simulink model "torque_to_theta"  (R2018b)
settings: Solver=FixedStepAuto  StartTime=0.0  StopTime=inf  RelTol=1e-3
values from neighbouring files (symbols this model uses):
  p = pi    (= 3.14159265359)    [nominal_model.m]
libraries: arduinolib x15, simulink x3
settings Model: ExtModeTrigDuration=2  Creator=paniz  LastModifiedBy=paniz
settings DataIOCC: ReturnWorkspaceOutputs=on
settings OptimizationCC: EnhancedBackFolding=on  PassReuseOutputArgsAs=Individual arguments  ZeroExternalMemoryAtStartup=off  ZeroInternalMemoryAtStartup=off  MaxStackSize=64  OptimizeBlockOrder=speed  DifferentSizesBufferReuse=on  OptimizationCustomize=off
settings DebuggingCC: ParameterTunabilityLossMsg=error  UnconnectedInputMsg=none  UnconnectedOutputMsg=none  UnconnectedLineMsg=none  SFMachineParentedDataDiag=error
settings HardwareCC: ProdBitPerInt=16  ProdBitPerPointer=16  ProdBitPerSizeT=16  ProdBitPerPtrDiffT=16  ProdLargestAtomicFloat=None  ProdWordSize=8  ProdHWDeviceType=Atmel->AVR
settings SFSimCC: MATLABDynamicMemAlloc=off
settings RTWCC: SystemTargetFile=ert.tlc  HardwareBoard=Arduino Mega 2560  TemplateMakefile=ert_default_tmf  Toolchain=Arduino AVR
settings CodeAppCC: ForceParamTrailComments=on  IgnoreCustomStorageClasses=off  OperatorAnnotations=on  SimulinkDataObjDesc=on  SFDataObjDesc=on  InsertBlockDesc=on
settings ERTTargetCC: SupportContinuousTime=on  SupportVariableSizeSignals=on  ExtMode=on  ExtModeTransport=3  ExtModeStaticAlloc=on  ExtModeStaticAllocSize=2048  ExtModeMexFile=ext_xcp  ExtModeMexArgs=0 5 921600 'C:\Users\paniz\myCodes\Using Arduino and Matlab\Codes\Simulink\3 Muscle with pressure regulator\untitled.elf' 3 1000  ExtModeIntrfLevel=Level2 - Open

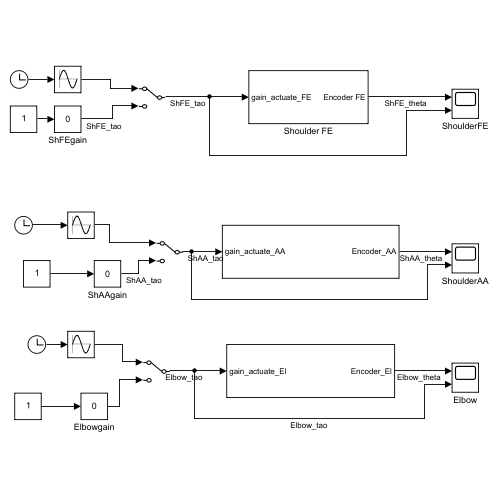
[thumbnail: Simulink's stored preview of the top-level diagram]
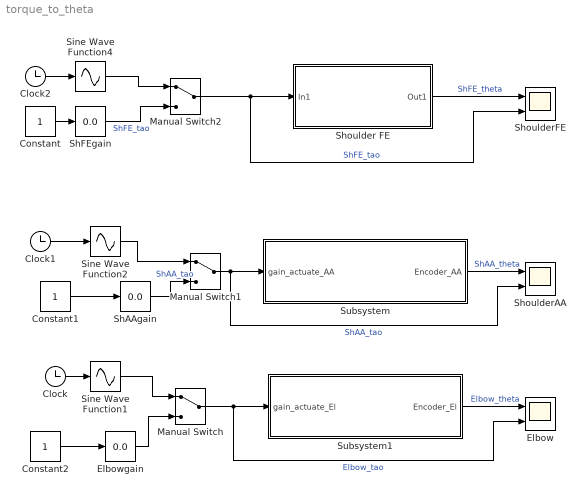
== system torque_to_theta ==
  Clock : Clock
  Clock1 : Clock
  Clock2 : Clock
  Constant : Constant
  Constant1 : Constant
  Constant2 : Constant
  Elbow : Scope  NumInputPorts=2
  Elbowgain : simulink/Math Operations/Slider Gain  gain=0.0  low=0  high=6
  Manual Switch : ManualSwitch
  Manual Switch1 : ManualSwitch
  Manual Switch2 : ManualSwitch
  ShAAgain : simulink/Math Operations/Slider Gain  gain=0.0  low=0  high=6
  ShFEgain : simulink/Math Operations/Slider Gain  gain=0.0  low=0  high=6
  Shoulder FE : Subsystem
  ShoulderAA : Scope  NumInputPorts=2
  ShoulderFE : Scope  NumInputPorts=2
  Sine Wave Function1 : Sin  TimeSource=Use external signal  Amplitude=2.3  Bias=2.30  Frequency=1/50  SampleTime=0
  Sine Wave Function2 : Sin  TimeSource=Use external signal  Amplitude=3  Bias=3  Frequency=1/50  Phase=-pi/3  SampleTime=0
  Sine Wave Function4 : Sin  TimeSource=Use external signal  Amplitude=3  Bias=3  Frequency=1/50  Phase=pi/6  SampleTime=0
  Subsystem : Subsystem
  Subsystem1 : Subsystem
  wires:
  Constant/1 -> ShFEgain/1
  ShFEgain/1 -> Manual Switch2/2  "ShFE_tao"
  Shoulder FE/1(Out1) -> ShoulderFE/1  "ShFE_theta"
  Manual Switch/1 -> Elbow/2, Subsystem1/1(gain_actuate_El)  "Elbow_tao"
  Subsystem1/1(Encoder_El) -> Elbow/1  "Elbow_theta"
  Subsystem/1(Encoder_AA) -> ShoulderAA/1  "ShAA_theta"
  Constant1/1 -> ShAAgain/1
  Constant2/1 -> Elbowgain/1
  Elbowgain/1 -> Manual Switch/2
  Sine Wave Function1/1 -> Manual Switch/1
  Clock/1 -> Sine Wave Function1/1
  Clock1/1 -> Sine Wave Function2/1
  Sine Wave Function2/1 -> Manual Switch1/1
  Manual Switch1/1 -> ShoulderAA/2, Subsystem/1(gain_actuate_AA)  "ShAA_tao"
  ShAAgain/1 -> Manual Switch1/2  "ShAA_tao"
  Clock2/1 -> Sine Wave Function4/1
  Sine Wave Function4/1 -> Manual Switch2/1
  Manual Switch2/1 -> ShoulderFE/2, Shoulder FE/1(In1)  "ShFE_tao"

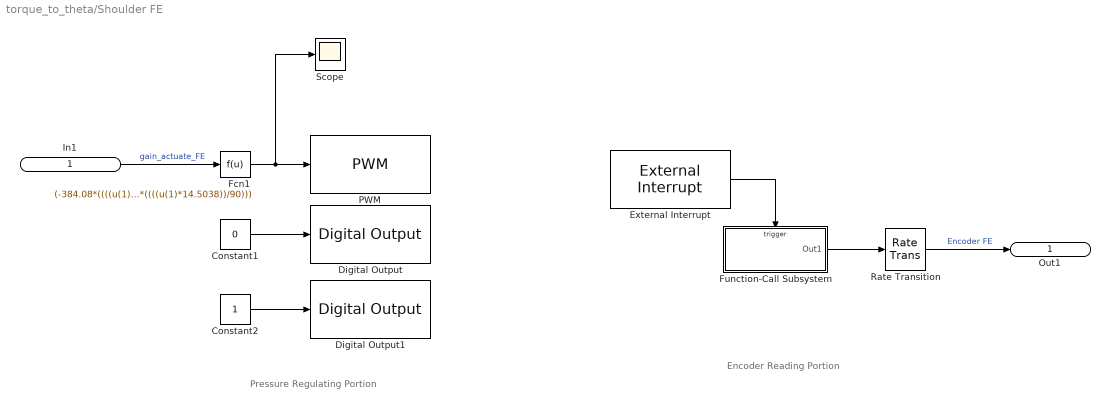
== system torque_to_theta/Shoulder FE ==
  note: Encoder Reading Portion
  note: Pressure Regulating Portion
  In1 : Inport
  Constant1 : Constant  Value=0  SampleTime=-1
  Constant2 : Constant  SampleTime=-1
  Digital Output : arduinolib/Digital Output  pinNumber=44  Direction=output  blockPlatform=arduino
  Digital Output1 : arduinolib/Digital Output  pinNumber=45  Direction=output  blockPlatform=arduino
  External Interrupt : arduinolib/External Interrupt  Pin=18  PullUp=off  Mode=RISING  InterruptSimulationInput=off
      settings: SourceProductBaseCode=ARDUINO
  Fcn1 : Fcn  Expr=(-384.08*((((u(1)*14.5038))/90))^4 + 789.52*((((u(1)*14.5038))/90))^3 - 618.81*((((u(1)*14.5038))/90))^2 + 468.18*((((u(1)*14.5038))/90)))
  Function-Call Subsystem : Subsystem  TreatAsAtomicUnit=on
  PWM : arduinolib/PWM  pinNumber=7  frequencyType=Specify  desiredFrequency=3921.16  achievableFrequency=3921.5686
  Rate Transition : RateTransition  Deterministic=off  OutPortSampleTimeOpt=Inherit
  Scope : Scope
  Out1 : Outport
  wires:
  Constant1/1 -> Digital Output/1
  Constant2/1 -> Digital Output1/1
  Function-Call Subsystem/1(Out1) -> Rate Transition/1
  Fcn1/1 -> Scope/1, PWM/1
  External Interrupt/1 -> Function-Call Subsystem/Trigger
  In1/1 -> Fcn1/1  "gain_actuate_FE"
  Rate Transition/1 -> Out1/1  "Encoder FE"

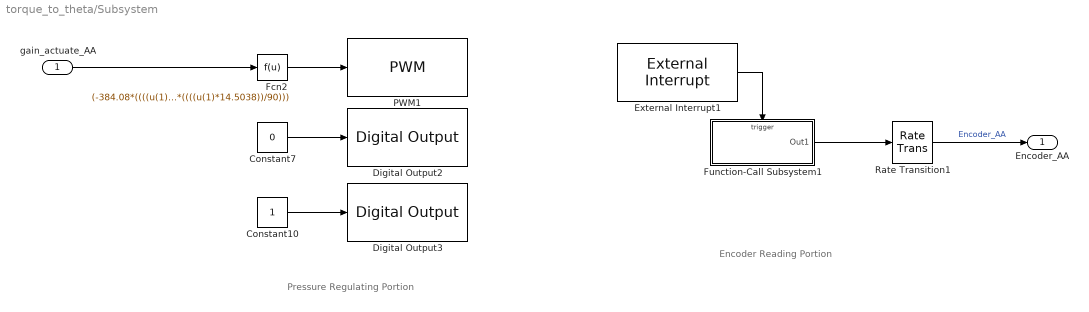
== system torque_to_theta/Subsystem ==
  note: Pressure Regulating Portion
  note: Encoder Reading Portion
  gain_actuate_AA : Inport
  Constant10 : Constant  SampleTime=-1
  Constant7 : Constant  Value=0  SampleTime=-1
  Digital Output2 : arduinolib/Digital Output  pinNumber=52  Direction=output  blockPlatform=arduino
  Digital Output3 : arduinolib/Digital Output  pinNumber=53  Direction=output  blockPlatform=arduino
  External Interrupt1 : arduinolib/External Interrupt  Pin=20  PullUp=off  Mode=RISING  InterruptSimulationInput=off
      settings: SourceProductBaseCode=ARDUINO
  Fcn2 : Fcn  Expr=(-384.08*((((u(1)*14.5038))/90))^4 + 789.52*((((u(1)*14.5038))/90))^3 - 618.81*((((u(1)*14.5038))/90))^2 + 468.18*((((u(1)*14.5038))/90)))
  Function-Call Subsystem1 : Subsystem  TreatAsAtomicUnit=on
  PWM1 : arduinolib/PWM  pinNumber=8  frequencyType=Specify  desiredFrequency=3921.16  achievableFrequency=3921.5686
  Rate Transition1 : RateTransition  Deterministic=off  OutPortSampleTimeOpt=Inherit
  Encoder_AA : Outport
  wires:
  Function-Call Subsystem1/1(Out1) -> Rate Transition1/1
  Constant7/1 -> Digital Output2/1
  Fcn2/1 -> PWM1/1
  Constant10/1 -> Digital Output3/1
  Rate Transition1/1 -> Encoder_AA/1  "Encoder_AA"
  External Interrupt1/1 -> Function-Call Subsystem1/Trigger
  gain_actuate_AA/1 -> Fcn2/1

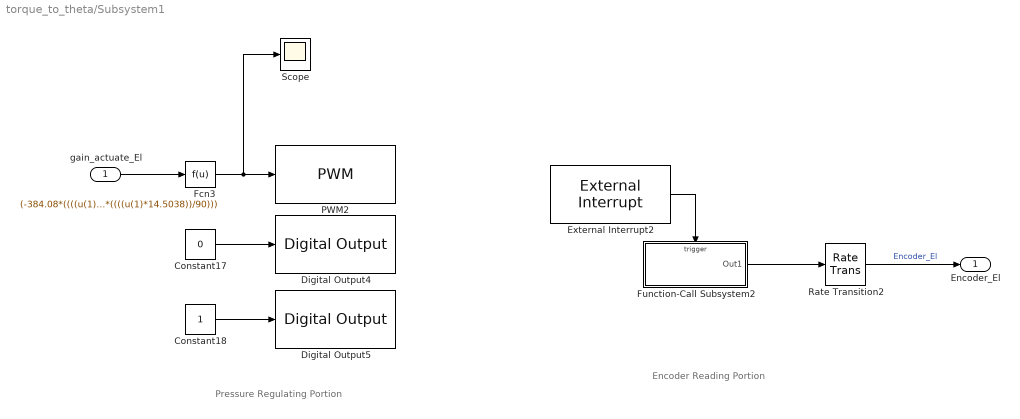
== system torque_to_theta/Subsystem1 ==
  note: Pressure Regulating Portion
  note: Encoder Reading Portion
  gain_actuate_El : Inport
  Constant17 : Constant  Value=0  SampleTime=-1
  Constant18 : Constant  SampleTime=-1
  Digital Output4 : arduinolib/Digital Output  pinNumber=17  Direction=output  blockPlatform=arduino
  Digital Output5 : arduinolib/Digital Output  pinNumber=5  Direction=output  blockPlatform=arduino
  External Interrupt2 : arduinolib/External Interrupt  Pin=3  PullUp=off  Mode=RISING  InterruptSimulationInput=off
      settings: SourceProductBaseCode=ARDUINO
  Fcn3 : Fcn  Expr=(-384.08*((((u(1)*14.5038))/90))^4 + 789.52*((((u(1)*14.5038))/90))^3 - 618.81*((((u(1)*14.5038))/90))^2 + 468.18*((((u(1)*14.5038))/90)))
  Function-Call Subsystem2 : Subsystem  TreatAsAtomicUnit=on
  PWM2 : arduinolib/PWM  pinNumber=6  frequencyType=Specify  desiredFrequency=3921.16  achievableFrequency=3921.5686
  Rate Transition2 : RateTransition  Deterministic=off  OutPortSampleTimeOpt=Inherit
  Scope : Scope
  Encoder_El : Outport
  wires:
  gain_actuate_El/1 -> Fcn3/1
  Fcn3/1 -> Scope/1, PWM2/1
  External Interrupt2/1 -> Function-Call Subsystem2/Trigger
  Function-Call Subsystem2/1(Out1) -> Rate Transition2/1
  Constant18/1 -> Digital Output5/1
  Constant17/1 -> Digital Output4/1
  Rate Transition2/1 -> Encoder_El/1  "Encoder_El"

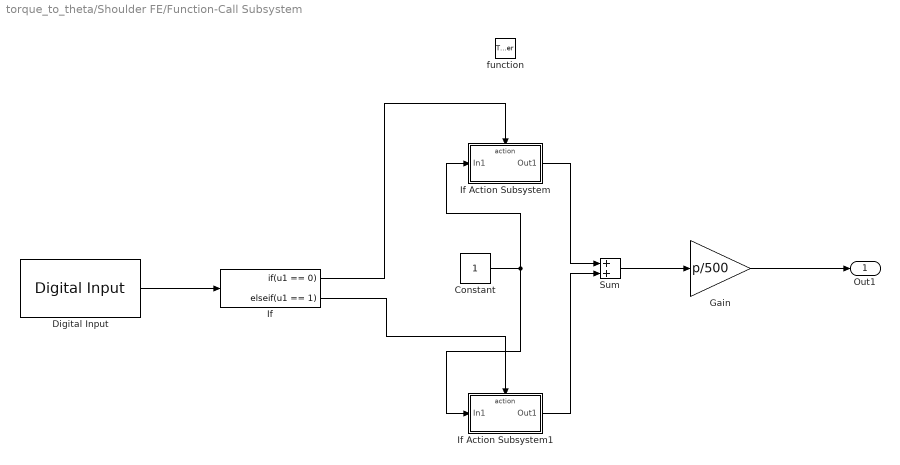
== system torque_to_theta/Shoulder FE/Function-Call Subsystem ==
  function : TriggerPort  TriggerType=function-call  VariantControl=Variant
  Constant : Constant
  Digital Input : arduinolib/Digital Input  pinNumber=19  mode=Default  Direction=input  SampleTime=-1  blockPlatform=arduino
  Gain : Gain  Gain=p/500
  If : If  IfExpression=u1 == 0  ElseIfExpressions=u1 == 1  ShowElse=off
  If Action Subsystem : Subsystem  TreatAsAtomicUnit=on
  If Action Subsystem1 : Subsystem  TreatAsAtomicUnit=on
  Sum : Sum
  Out1 : Outport
  wires:
  If/1 -> If Action Subsystem/Action
  If/2 -> If Action Subsystem1/Action
  Constant/1 -> If Action Subsystem1/1(In1), If Action Subsystem/1(In1)
  If Action Subsystem/1(Out1) -> Sum/1
  Sum/1 -> Gain/1
  If Action Subsystem1/1(Out1) -> Sum/2
  Digital Input/1 -> If/1
  Gain/1 -> Out1/1

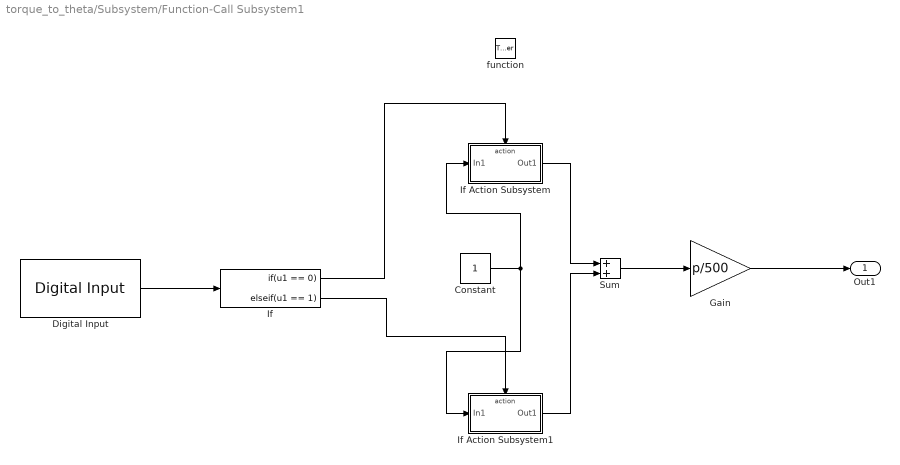
== system torque_to_theta/Subsystem/Function-Call Subsystem1 ==
  function : TriggerPort  TriggerType=function-call  VariantControl=Variant
  Constant : Constant
  Digital Input : arduinolib/Digital Input  pinNumber=21  mode=Default  Direction=input  SampleTime=-1  blockPlatform=arduino
  Gain : Gain  Gain=p/500
  If : If  IfExpression=u1 == 0  ElseIfExpressions=u1 == 1  ShowElse=off
  If Action Subsystem : Subsystem  TreatAsAtomicUnit=on
  If Action Subsystem1 : Subsystem  TreatAsAtomicUnit=on
  Sum : Sum
  Out1 : Outport
  wires:
  If/1 -> If Action Subsystem/Action
  If/2 -> If Action Subsystem1/Action
  Constant/1 -> If Action Subsystem1/1(In1), If Action Subsystem/1(In1)
  If Action Subsystem/1(Out1) -> Sum/1
  Sum/1 -> Gain/1
  If Action Subsystem1/1(Out1) -> Sum/2
  Digital Input/1 -> If/1
  Gain/1 -> Out1/1

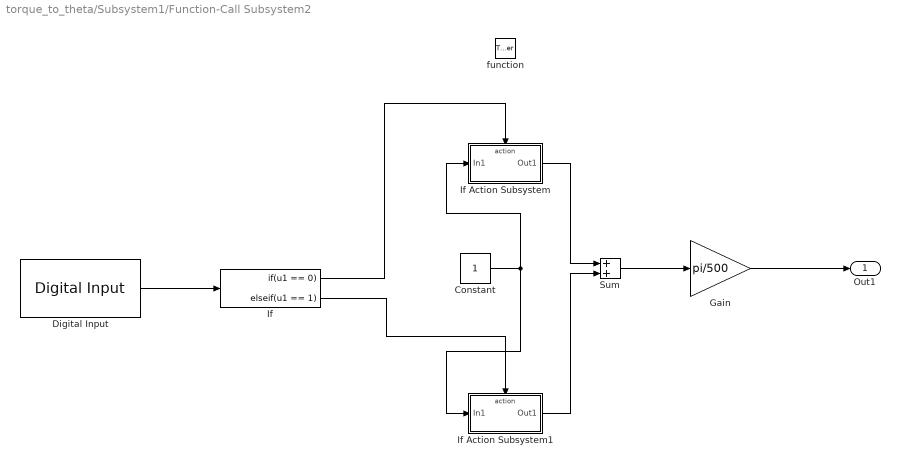
== system torque_to_theta/Subsystem1/Function-Call Subsystem2 ==
  function : TriggerPort  TriggerType=function-call  VariantControl=Variant
  Constant : Constant
  Digital Input : arduinolib/Digital Input  pinNumber=2  mode=Default  Direction=input  SampleTime=-1  blockPlatform=arduino
  Gain : Gain  Gain=pi/500
  If : If  IfExpression=u1 == 0  ElseIfExpressions=u1 == 1  ShowElse=off
  If Action Subsystem : Subsystem  TreatAsAtomicUnit=on
  If Action Subsystem1 : Subsystem  TreatAsAtomicUnit=on
  Sum : Sum
  Out1 : Outport
  wires:
  If/1 -> If Action Subsystem/Action
  If/2 -> If Action Subsystem1/Action
  Constant/1 -> If Action Subsystem1/1(In1), If Action Subsystem/1(In1)
  If Action Subsystem/1(Out1) -> Sum/1
  Sum/1 -> Gain/1
  If Action Subsystem1/1(Out1) -> Sum/2
  Digital Input/1 -> If/1
  Gain/1 -> Out1/1

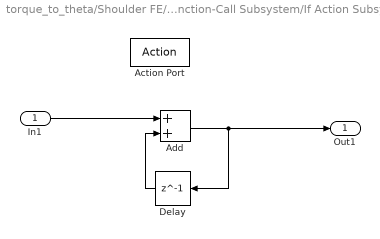
== system torque_to_theta/Shoulder FE/Function-Call Subsystem/If Action Subsystem ==
  In1 : Inport
  Action Port : ActionPort
  Add : Sum
  Delay : Delay  DelayLength=1
  Out1 : Outport
  wires:
  Add/1 -> Delay/1, Out1/1
  Delay/1 -> Add/2
  In1/1 -> Add/1

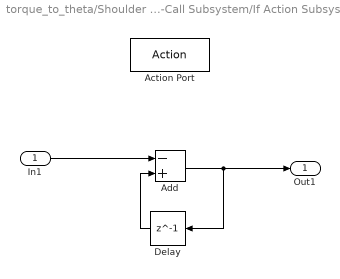
== system torque_to_theta/Shoulder FE/Function-Call Subsystem/If Action Subsystem1 ==
  In1 : Inport
  Action Port : ActionPort
  Add : Sum  Inputs=-+
  Delay : Delay  DelayLength=1
  Out1 : Outport
  wires:
  Delay/1 -> Add/2
  Add/1 -> Delay/1, Out1/1
  In1/1 -> Add/1

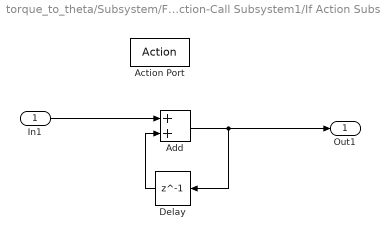
== system torque_to_theta/Subsystem/Function-Call Subsystem1/If Action Subsystem ==
  In1 : Inport
  Action Port : ActionPort
  Add : Sum
  Delay : Delay  DelayLength=1
  Out1 : Outport
  wires:
  Add/1 -> Delay/1, Out1/1
  Delay/1 -> Add/2
  In1/1 -> Add/1

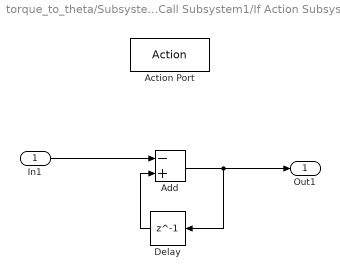
== system torque_to_theta/Subsystem/Function-Call Subsystem1/If Action Subsystem1 ==
  In1 : Inport
  Action Port : ActionPort
  Add : Sum  Inputs=-+
  Delay : Delay  DelayLength=1
  Out1 : Outport
  wires:
  Delay/1 -> Add/2
  Add/1 -> Delay/1, Out1/1
  In1/1 -> Add/1

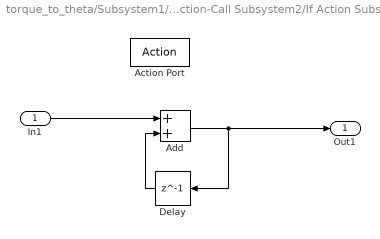
== system torque_to_theta/Subsystem1/Function-Call Subsystem2/If Action Subsystem ==
  In1 : Inport
  Action Port : ActionPort
  Add : Sum
  Delay : Delay  DelayLength=1
  Out1 : Outport
  wires:
  Add/1 -> Delay/1, Out1/1
  Delay/1 -> Add/2
  In1/1 -> Add/1

== system torque_to_theta/Subsystem1/Function-Call Subsystem2/If Action Subsystem1 ==
  In1 : Inport
  Action Port : ActionPort
  Add : Sum  Inputs=-+
  Delay : Delay  DelayLength=1
  Out1 : Outport
  wires:
  Delay/1 -> Add/2
  Add/1 -> Delay/1, Out1/1
  In1/1 -> Add/1
